simulink model "Copter_Plane_h3zh_sl_4a1rh"  (R2020b)
(part 2 of 3)

  use_sqrt_controller1 : DataStoreMemory  DataStoreName=use_sqrt_controller  ReadBeforeWriteMsg=warning  WriteAfterWriteMsg=warning  WriteAfterReadMsg=warning  InitialValue=use_sqrt_controller  ShowAdditionalParam=off  OutDataTypeStr=double
  vdot_filter1 : DataStoreMemory  DataStoreName=vdot_filter  ReadBeforeWriteMsg=warning  WriteAfterWriteMsg=warning  WriteAfterReadMsg=warning  InitialValue=vdot_filter  ShowAdditionalParam=off  OutDataTypeStr=double
  vel_desired1 : DataStoreMemory  DataStoreName=vel_desired  ReadBeforeWriteMsg=warning  WriteAfterWriteMsg=warning  WriteAfterReadMsg=warning  InitialValue=vel_desired  VectorParams1D=off  ShowAdditionalParam=off  OutDataTypeStr=double
  vel_dot1 : DataStoreMemory  DataStoreName=vel_dot  ReadBeforeWriteMsg=warning  WriteAfterWriteMsg=warning  WriteAfterReadMsg=warning  InitialValue=vel_dot  VectorParams1D=off  ShowAdditionalParam=off  OutDataTypeStr=double
  vel_error1 : DataStoreMemory  DataStoreName=vel_error  ReadBeforeWriteMsg=warning  WriteAfterWriteMsg=warning  WriteAfterReadMsg=warning  InitialValue=vel_error  VectorParams1D=off  ShowAdditionalParam=off  OutDataTypeStr=double
  vel_error_input1 : DataStoreMemory  DataStoreName=vel_error_input  ReadBeforeWriteMsg=warning  WriteAfterWriteMsg=warning  WriteAfterReadMsg=warning  InitialValue=vel_error_input  VectorParams1D=off  ShowAdditionalParam=off  OutDataTypeStr=double
  vel_forward_gain1 : DataStoreMemory  DataStoreName=vel_forward_gain  ReadBeforeWriteMsg=warning  WriteAfterWriteMsg=warning  WriteAfterReadMsg=warning  InitialValue=vel_forward_gain  VectorParams1D=off  ShowAdditionalParam=off  OutDataTypeStr=double
  vel_forward_integrator : DataStoreMemory  DataStoreName=vel_forward_integrator  ReadBeforeWriteMsg=warning  WriteAfterWriteMsg=warning  WriteAfterReadMsg=warning  InitialValue=vel_forward_integrator  VectorParams1D=off  ShowAdditionalParam=off  OutDataTypeStr=double
  vel_forward_last_pct1 : DataStoreMemory  DataStoreName=vel_forward_last_pct  ReadBeforeWriteMsg=warning  WriteAfterWriteMsg=warning  WriteAfterReadMsg=warning  InitialValue=vel_forward_last_pct  VectorParams1D=off  ShowAdditionalParam=off  OutDataTypeStr=double
  vel_forward_min_pitch1 : DataStoreMemory  DataStoreName=vel_forward_min_pitch  ReadBeforeWriteMsg=warning  WriteAfterWriteMsg=warning  WriteAfterReadMsg=warning  InitialValue=vel_forward_min_pitch  VectorParams1D=off  ShowAdditionalParam=off  OutDataTypeStr=double
  vel_forward_tail_tilt_max1 : DataStoreMemory  DataStoreName=vel_forward_tail_tilt_max  ReadBeforeWriteMsg=warning  WriteAfterWriteMsg=warning  WriteAfterReadMsg=warning  InitialValue=vel_forward_tail_tilt_max  VectorParams1D=off  ShowAdditionalParam=off  OutDataTypeStr=double
  vel_last1 : DataStoreMemory  DataStoreName=vel_last  ReadBeforeWriteMsg=warning  WriteAfterWriteMsg=warning  WriteAfterReadMsg=warning  InitialValue=vel_last  VectorParams1D=off  ShowAdditionalParam=off  OutDataTypeStr=double
  vel_target1 : DataStoreMemory  DataStoreName=vel_target  ReadBeforeWriteMsg=warning  WriteAfterWriteMsg=warning  WriteAfterReadMsg=warning  InitialValue=vel_target  VectorParams1D=off  ShowAdditionalParam=off  OutDataTypeStr=double
  vertAccLim1 : DataStoreMemory  DataStoreName=vertAccLim  ReadBeforeWriteMsg=warning  WriteAfterWriteMsg=warning  WriteAfterReadMsg=warning  InitialValue=vertAccLim  VectorParams1D=off  ShowAdditionalParam=off  OutDataTypeStr=double
  weathervane_gain1 : DataStoreMemory  DataStoreName=weathervane_gain  ReadBeforeWriteMsg=warning  WriteAfterWriteMsg=warning  WriteAfterReadMsg=warning  InitialValue=weathervane_gain  VectorParams1D=off  ShowAdditionalParam=off  OutDataTypeStr=double
  weathervane_last_output1 : DataStoreMemory  DataStoreName=weathervane_last_output  ReadBeforeWriteMsg=warning  WriteAfterWriteMsg=warning  WriteAfterReadMsg=warning  InitialValue=weathervane_last_output  VectorParams1D=off  ShowAdditionalParam=off  OutDataTypeStr=double
  weathervane_min_roll1 : DataStoreMemory  DataStoreName=weathervane_min_roll  ReadBeforeWriteMsg=warning  WriteAfterWriteMsg=warning  WriteAfterReadMsg=warning  InitialValue=weathervane_min_roll  VectorParams1D=off  ShowAdditionalParam=off  OutDataTypeStr=double
  yaw1 : DataStoreMemory  DataStoreName=yaw  ReadBeforeWriteMsg=warning  WriteAfterWriteMsg=warning  WriteAfterReadMsg=warning  InitialValue=yaw  VectorParams1D=off  ShowAdditionalParam=off  OutDataTypeStr=double
  yaw_factor1 : DataStoreMemory  DataStoreName=yaw_factor  ReadBeforeWriteMsg=warning  WriteAfterWriteMsg=warning  WriteAfterReadMsg=warning  InitialValue=yaw_factor  VectorParams1D=off  ShowAdditionalParam=off  OutDataTypeStr=double
  yaw_headroom1 : DataStoreMemory  DataStoreName=yaw_headroom  ReadBeforeWriteMsg=warning  WriteAfterWriteMsg=warning  WriteAfterReadMsg=warning  InitialValue=yaw_headroom  VectorParams1D=off  ShowAdditionalParam=off  OutDataTypeStr=double
  yaw_in1 : DataStoreMemory  DataStoreName=yaw_in  ReadBeforeWriteMsg=warning  WriteAfterWriteMsg=warning  WriteAfterReadMsg=warning  InitialValue=yaw_in  VectorParams1D=off  ShowAdditionalParam=off  OutDataTypeStr=double
  yaw_in_max : DataStoreMemory  DataStoreName=yaw_in_max  ReadBeforeWriteMsg=warning  WriteAfterWriteMsg=warning  WriteAfterReadMsg=warning  InitialValue=yaw_in_max  VectorParams1D=off  ShowAdditionalParam=off  OutDataTypeStr=double
  yaw_max_c2p1 : DataStoreMemory  DataStoreName=yaw_max_c2p  ReadBeforeWriteMsg=warning  WriteAfterWriteMsg=warning  WriteAfterReadMsg=warning  InitialValue=yaw_max_c2p  VectorParams1D=off  ShowAdditionalParam=off  OutDataTypeStr=double
  yaw_rate_max1 : DataStoreMemory  DataStoreName=yaw_rate_max  ReadBeforeWriteMsg=warning  WriteAfterWriteMsg=warning  WriteAfterReadMsg=warning  InitialValue=yaw_rate_max  VectorParams1D=off  ShowAdditionalParam=off  OutDataTypeStr=double
  yaw_t1 : Lookup_n-D  NumberOfTableDimensions=1  BreakpointsForDimension1=time_algo  Table=algo_yaw  InternalRulePriority=Speed  RndMeth=Simplest  InputSameDT=on
  z_accel_meas1 : DataStoreMemory  DataStoreName=z_accel_meas  ReadBeforeWriteMsg=warning  WriteAfterWriteMsg=warning  WriteAfterReadMsg=warning  InitialValue=z_accel_meas  VectorParams1D=off  ShowAdditionalParam=off  OutDataTypeStr=double
  Out1 : Outport  OutDataTypeStr=Bus: BUS_CTRL_Sevro_pwm
  wires:
  Gain15/1 -> Scope89/1
  Data Store Read75/1 -> Gain15/1
  Data Store Read77/1 -> Gain17/1
  Gain16/1 -> Scope90/1
  Data Store Read76/1 -> Gain16/1
  Gain17/1 -> Scope91/1
  Data Store Read2/1 -> Scope10/1
  Gain8/1 -> Scope13/1
  Gain3/1 -> Scope12/1
  Gain2/1 -> Scope11/1
  Data Store Read3/1 -> Gain2/1
  Data Store Read4/1 -> Gain3/1
  Data Store Read35/1 -> Gain8/1
  Data Store Read47/1 -> Demux/1
  Demux/1 -> Scope24/1
  Demux/2 -> Scope24/2
  Demux17/3 -> Scope14/3
  Demux17/2 -> Scope14/2
  Demux17/1 -> Scope14/1
  Data Store Read78/1 -> Demux17/1
  Data Store Read82/1 -> Scope39/1
  Data Store Read81/1 -> Scope30/1
  Data Store Read80/1 -> Scope23/1
  Data Store Read49/1 -> Scope47/1
  Data Store Read89/1 -> Scope63/1
  Data Store Read91/1 -> Scope69/1
  Data Store Read94/1 -> Scope6/2
  Data Store Read96/1 -> Scope16/2
  Data Store Read93/1 -> Scope18/2
  Data Store Read95/1 -> Scope132/1, Scope19/2
  Data Store Read97/1 -> Scope82/1
  Data Store Read98/1 -> Scope84/1
  Data Store Read99/1 -> Gain21/1
  Gain21/1 -> Scope107/2
  Data Store Read100/1 -> Gain22/1
  Gain22/1 -> Scope34/1, Scope4/1, Scope107/1
  Gain25/1 -> Scope35/1, Scope111/1
  Gain24/1 -> Scope111/2
  Data Store Read104/1 -> Gain24/1
  Data Store Read103/1 -> Scope36/1, Gain25/1
  Data Store Read105/1 -> Scope112/1
  Data Store Read106/1 -> Scope112/2
  Data Store Read5/1 -> Scope3/2, Scope1/1
  Data Store Read6/1 -> Scope3/1, Scope2/1
  Data Store Read8/1 -> Scope5/2
  Data Store Read7/1 -> Scope5/1, Scope4/2
  Data Store Read10/1 -> Scope8/1
  Data Store Read12/1 -> Scope109/1, Scope9/1
  Data Store Read13/1 -> Scope9/2
  Data Store Read14/1 -> Gain1/1
  Gain1/1 -> Scope8/2
  Data Store Read9/1 -> Scope15/1
  algo_throttle_dem/1 -> Data Store Write3/1
  Clock1/1 -> algo_pitch_dem/1, algo_k_aileron/1, algo_k_throttle/1, algo_k_rudder/1, algo_k_elevator/1
  algo_k_aileron/1 -> Gain61/1
  algo_k_elevator/1 -> Gain62/1
  algo_k_rudder/1 -> Gain63/1
  algo_k_throttle/1 -> Gain26/1
  Data Store Read17/1 -> Gain13/1
  Gain12/1 -> Scope41/3
  Gain13/1 -> Scope41/4
  Data Store Read16/1 -> Scope41/2, Scope42/2, Scope40/1
  Data Store Read/1 -> Scope42/1, Scope41/1, Scope/1
  Data Store Read15/1 -> Gain12/1
  Data Store Read18/1 -> Gain14/1
  Gain14/1 -> Scope112/3
  Data Store Read19/1 -> Scope43/1
  Data Store Read20/1 -> Scope43/2
  EAS_Algo/1 -> ?
  algo_curr_alt_0/1 -> Data Store Write19/1
  algo_curVelNED_2/1 -> Data Store Write25/1
  Data Store Read21/1 -> Gain18/1
  algo_pitch_dem/1 -> Scope38/1
  Gain18/1 -> Scope38/2
  Data Store Read23/1 -> Scope45/1
  Mux1/1 -> Gain69/1
  Gain30/1 -> Data Store Write30/1
  Gain32/1 -> Data Store Write42/1
  algo_remote_ct_st_throttle/1 -> Data Store Write40/1
  algo_roll_target_pilot/1 -> Gain10/1
  gx_f2/1 -> Gain19/1
  algo_current_loc_1/1 -> Mux2/2
  algo_curr_vel_2/1 -> Mux1/3
  algo_pitch_target_pilot/1 -> Gain11/1
  algo_remote_ct_st_yaw/1 -> Data Store Write45/1
  gy_f2/1 -> Gain32/1
  pitch_t1/1 -> Gain29/1
  algo_remote_ct_st_pitch/1 -> Data Store Write35/1
  ay_f2/1 -> Data Store Write31/1
  az_f2/1 -> Data Store Write36/1
  algo_curr_vel_0/1 -> Mux1/1
  algo_climb_rate_cms/1 -> Gain65/1
  algo_curr_vel_1/1 -> Mux1/2
  algo_curr_alt/1 -> Gain64/1
  ax_f2/1 -> Data Store Write32/1
  gz_f2/1 -> Gain33/1
  roll_t1/1 -> Gain30/1
  yaw_t1/1 -> Gain31/1
  Gain19/1 -> Data Store Write41/1
  Gain31/1 -> Data Store Write39/1
  Mux2/1 -> Gain/1
  Gain33/1 -> Data Store Write43/1
  algo_current_loc_0/1 -> Mux2/1
  Gain29/1 -> Data Store Write38/1
  algo_remote_ct_st_roll/1 -> Data Store Write8/1
  algo_curVelNED_1/1 -> Data Store Write5/1
  algo_curVelNED_0/1 -> Data Store Write4/1
  algo_throttle_upper/1 -> Scope66/1
  Data Store Read51/1 -> Demux1/1
  Data Store Read28/1 -> Scope58/2
  algo_rate_target_ang_vel_0/1 -> Gain6/1
  algo_z_accel_meas/1 -> Gain71/1
  algo_pos_target_0/1 -> Scope31/1
  Data Store Read33/1 -> Gain73/1
  Data Store Read53/1 -> Scope110/1, Scope37/2
  Data Store Read52/1 -> Scope32/2
  Data Store Read11/1 -> Gain53/1
  Data Store Read37/1 -> Gain89/1
  Data Store Read45/1 -> Gain4/1
  algo_vel_target_0/1 -> Scope25/1
  Clock5/1 -> algo_curr_pos_1/1, algo_curr_pos_0/1
  Gain5/1 -> Data Store Write7/1, Scope65/1
  Data Store Read50/1 -> Scope65/3
  algo_vel_desired_2/1 -> Scope26/1
  Gain6/1 -> Data Store Write/1, Scope59/1
  algo_rate_target_ang_vel_1/1 -> Gain7/1
  Demux1/1 -> Scope44/2
  algo_curr_pos_0/1 -> Scope44/1
  Clock6/1 -> algo_rate_target_ang_vel_2/1, algo_rate_target_ang_vel_1/1, algo_rate_target_ang_vel_0/1
  Data Store Read54/1 -> Scope60/2
  Demux1/2 -> Scope27/2
  Gain37/1 -> Scope61/1
  algo_vel_target_2/1 -> Gain66/1
  Clock12/1 -> algo_pitch_in/1
  algo_pos_target_1/1 -> Scope20/1
  Clock9/1 -> algo_roll_in/1
  Gain40/1 -> Scope64/2
  Data Store Read30/1 -> Scope56/2, Scope48/1
  Clock13/1 -> algo_yaw_in/1
  Clock3/1 -> algo_vel_target_1/1, algo_accel_target_1/1, algo_pos_target_1/1
  Clock10/1 -> algo_throttle_filter/1
  Data Store Read31/1 -> Scope29/2
  Data Store Read46/1 -> Scope59/3
  Data Store Read26/1 -> Derivative/1, Scope21/2
  algo_vel_target_1/1 -> Scope67/1
  Data Store Read44/1 -> Gain40/1
  Data Store Read25/1 -> Gain86/1
  Data Store Read42/1 -> Gain37/1
  Data Store Read24/1 -> Gain88/1
  Data Store Read22/1 -> Scope62/2, Scope110/2
  Data Store Read36/1 -> Gain91/1
  Gain39/1 -> Scope61/2
  Clock11/1 -> algo_pwm_out_4/1, algo_pwm_out_3/1, algo_pwm_out_2/1, algo_pwm_out_1/1
  Data Store Read43/1 -> Gain39/1
  Data Store Read1/1 -> Scope59/2
  algo_roll_in/1 -> Gain48/1
  algo_pwm_out_1/1 -> Scope46/1
  Data Store Read32/1 -> Scope33/2
  Data Store Read55/1 -> Scope65/2
  Clock8/1 -> algo_pos_target_0/1, algo_accel_target_0/1, algo_vel_target_0/1
  algo_pwm_out_2/1 -> Scope49/1
  algo_accel_target_1/1 -> Scope68/1
  Data Store Read29/1 -> Scope66/2
  algo_accel_target_2/1 -> Gain70/1
  Clock4/1 -> algo_throttle_upper/1, algo_throttle_lower/1, algo_limit_pos_up/1
  algo_throttle_lower/1 -> Scope58/1
  Clock7/1 -> algo_pos_target_2/1, algo_z_accel_meas/1, algo_accel_target_2/1, algo_vel_target_2/1, algo_vel_desired_2/1
  algo_yaw_in/1 -> Gain93/1
  algo_accel_target_0/1 -> Scope28/1
  algo_pitch_in/1 -> Gain92/1
  algo_limit_pos_up/1 -> Scope56/1
  algo_rate_target_ang_vel_2/1 -> Gain5/1
  Data Store Read41/1 -> Scope55/2
  Data Store Read38/1 -> Scope46/2
  Data Store Read34/1 -> Gain90/1
  Gain4/1 -> Scope64/1
  algo_curr_pos_1/1 -> Scope27/1
  algo_throttle_filter/1 -> Gain27/1
  algo_pwm_out_4/1 -> Scope55/1
  Data Store Read40/1 -> Scope50/2
  Data Store Read27/1 -> Derivative1/1, Scope22/2
  Data Store Read39/1 -> Scope49/2
  algo_pwm_out_3/1 -> Scope50/1
  Data Store Read48/1 -> Scope60/3
  Data Store Read56/1 -> Gain87/1
  Data Store Read57/1 -> Demux2/1
  Demux2/1 -> Scope17/1
  Demux2/2 -> Scope17/2
  Demux2/3 -> Scope17/3
  Gain7/1 -> Data Store Write6/1, Scope60/1
  algo_tail_tilt/1 -> Gain9/1
  Gain9/1 -> Data Store Write9/1
  Gain/1 -> Data Store Write33/1
  Gain10/1 -> Data Store Write34/1
  Gain11/1 -> Data Store Write37/1
  Data Store Read58/1 -> Demux3/1
  Data Store Read60/1 -> Scope53/1
  Demux3/1 -> Gain23/1
  Gain23/1 -> Scope53/2
  Demux3/2 -> Gain28/1
  Gain28/1 -> Scope70/1
  Data Store Read59/1 -> Scope70/2
  Data Store Read61/1 -> Scope71/1
  Data Store Read62/1 -> Scope71/2
  Data Store Read63/1 -> Scope72/2
  Data Store Read64/1 -> Scope52/1
  Data Store Read65/1 -> Scope71/3, Scope72/1
  EAS2TAS_Algo/1 -> Data Store Write18/1
  Gain34/1 -> Scope76/1
  Data Store Read69/1 -> Scope76/2
  Data Store Read68/1 -> Gain34/1
  Clock14/1 -> algo_weathervane_last_output/1
  algo_weathervane_last_output/1 -> Scope77/1
  Data Store Read70/1 -> Scope77/2
  Clock15/1 -> algo_attitude_target_euler_angle_2/1, algo_attitude_target_euler_angle_1/1, algo_attitude_target_euler_angle_0/1
  Data Store Read73/1 -> Gain35/1
  algo_attitude_target_euler_angle_2/1 -> Scope51/1
  Gain35/1 -> Scope51/2
  Data Store Read90/1 -> Scope87/1
  Data Store Read88/1 -> Scope87/2
  Data Store Read92/1 -> Scope88/2
  Data Store Read101/1 -> Scope88/1
  algo_flightTaskMode/1 -> Scope141/1, Data Type Conversion/1
  Data Type Conversion/1 -> Data Store Write12/1
  Data Store Read120/1 -> Demux4/1
  Data Store Read121/1 -> Gain49/1
  algo_attitude_target_euler_angle_1/1 -> Scope102/1
  Data Store Read124/1 -> Gain50/1
  algo_attitude_target_euler_angle_0/1 -> Scope103/1
  Gain49/1 -> Scope102/2
  Gain50/1 -> Scope103/2
  Data Store Read126/1 -> Scope105/2
  Data Store Read125/1 -> Scope104/2
  algo_attitude_target_euler_rate_0/1 -> Scope105/1
  algo_attitude_target_euler_rate_1/1 -> Scope104/1
  Data Store Read127/1 -> Scope106/2
  algo_attitude_target_euler_rate_2/1 -> Scope106/1
  Clock19/1 -> algo_attitude_target_euler_rate_0/1, algo_attitude_target_euler_rate_1/1, algo_attitude_target_euler_rate_2/1
  Data Store Read129/1 -> Gain51/1
  Gain51/1 -> Scope108/1, Scope109/2
  Data Store Read128/1 -> Scope108/2
  algo_heightCmd/1 -> Gain52/1
  Gain52/1 -> Data Store Write11/1
  algo_maxClimbSpeed/1 -> Data Store Write13/1
  algo_pos_target_2/1 -> Scope136/3, Scope7/1
  algo_turnCenterLL_0/1 -> Gain55/1
  algo_turnCenterLL_1/1 -> Gain56/1
  Gain55/1 -> Data Store Write14/1
  Gain56/1 -> Data Store Write15/1
  algo_prePathPoint_LLA_0/1 -> Gain57/1
  Gain57/1 -> Data Store Write16/1
  algo_prePathPoint_LLA_1/1 -> Gain58/1
  Gain58/1 -> Data Store Write17/1
  algo_curPathPoint_LLA_0/1 -> Gain59/1
  Gain59/1 -> Data Store Write20/1
  Gain60/1 -> Data Store Write21/1
  algo_curPathPoint_LLA_1/1 -> Gain60/1
  Gain61/1 -> Scope6/1
  Gain62/1 -> Scope16/1
  Gain63/1 -> Scope18/1
  Gain64/1 -> Data Store Write44/1
  Gain65/1 -> Data Store Write26/1
  Gain66/1 -> Scope32/1
  Data Store Read130/1 -> Scope115/1
  Clock16/1 -> algo_hgt_dem/1
  Data Store Read131/1 -> Gain67/1
  algo_hgt_dem/1 -> Scope116/1
  Gain67/1 -> Scope116/2
  Clock20/1 -> algo_nav_roll/1
  algo_nav_roll/1 -> Scope117/1
  Data Store Read132/1 -> Gain68/1
  Gain68/1 -> Scope117/2
  Clock21/1 -> algo_latAccDem1/1
  algo_latAccDem1/1 -> Scope118/1
  Data Store Read133/1 -> Scope118/2
  Data Store Read137/1 -> Scope122/1
  algo_nav_pitch_cd/1 -> Scope122/2, Data Store Write2/1
  algo_rollCmd/1 -> Data Store Write22/1
  Data Store Read138/1 -> Scope57/1
  Clock22/1 -> algo_curPosNED_1/1, algo_curPosNED_0/1
  Data Store Read140/1 -> Demux6/1
  Data Store Read141/1 -> Demux5/1
  Data Store Read139/1 -> Demux7/1
  Demux6/1 -> Scope123/1  "pre"
  Demux5/1 -> Scope123/2  "net"
  Demux6/2 -> Scope124/1
  Demux5/2 -> Scope124/2
  Demux7/2 -> Scope127/1, Scope124/3  "cur"
  algo_curPosNED_0/1 -> ?
  algo_curPosNED_1/1 -> ?
  Gain69/1 -> Data Store Write46/1
  Gain70/1 -> Scope37/1
  Gain71/1 -> Scope62/1
  Gain73/1 -> Scope26/2
  Gain53/1 -> Scope7/2
  algo_pos_target_2a/1 -> Gain75/1
  algo_vel_desired_2a/1 -> Gain74/1
  Gain74/1 -> Data Store Write24/1
  Gain75/1 -> Data Store Write23/1
  Data Store Read152/1 -> Scope130/1
  Data Store Read153/1 -> Scope131/1
  algo_arspeed/1 -> Scope131/2
  Clock23/1 -> algo_arspeed/1
  Data Store Read154/1 -> Scope133/1, Scope132/2
  Data Store Read155/1 -> Scope133/2
  Data Store Read157/1 -> Gain80/1
  Gain80/1 -> Scope134/2
  Data Store Read156/1 -> Scope134/1
  Gain81/1 -> Scope136/1
  Data Store Read162/1 -> Gain81/1
  Data Store Read163/1 -> Gain82/1
  Gain82/1 -> Scope136/2
  Data Store Read164/1 -> Scope137/1
  Data Store Read168/1 -> Demux8/1
  Demux8/1 -> Scope126/2  "cur"
  Demux7/1 -> Scope126/1, Scope123/3
  Demux8/2 -> Scope127/2  "cur"
  Gain86/1 -> Scope20/2
  Gain87/1 -> Scope67/2
  Gain88/1 -> Scope68/2
  Gain89/1 -> Scope31/2
  Gain90/1 -> Scope25/2
  Gain91/1 -> Scope28/2
  Clock17/1 -> algo_tail_tilt1/1
  algo_tail_tilt1/1 -> Scope101/2
  Data Store Read170/1 -> Scope101/1
  Clock24/1 -> algo_throttle_dem1/1
  algo_throttle_dem1/1 -> Scope139/1
  Data Store Read66/1 -> Scope139/2
  Data Store Read169/1 -> Scope140/1
  algo_plane_mode/1 -> Data Type Conversion1/1
  Data Type Conversion1/1 -> Data Store Write27/1, Scope142/1
  algo_flightControlMode/1 -> Data Type Conversion2/1
  Data Type Conversion2/1 -> Scope143/1, Data Store Write28/1
  algo_mode/1 -> Scope113/1, Ceil1/1
  Ceil1/1 -> Scope114/1, Data Store Write29/1
  Clock2/1 -> algo_hgt_dem1/1, algo_tail_tilt/1, yaw_t1/1, roll_t1/1, pitch_t1/1, gz_f2/1, gy_f2/1, gx_f2/1, az_f2/1, ay_f2/1, ax_f2/1, algo_current_loc_1/1, algo_current_loc_0/1, algo_curr_alt_0/1, algo_curr_alt/1, algo_curr_vel_1/1, algo_curVelNED_2/1, algo_curVelNED_0/1, EAS_Algo/1, EAS2TAS_Algo/1, algo_pitch_target_pilot/1, algo_roll_target_pilot/1, algo_climb_rate_cms/1, algo_remote_ct_st_roll/1, algo_remote_ct_st_throttle/1, algo_mode/1, algo_nav_pitch_cd/1, algo_plane_mode/1, algo_turnCenterLL_1/1, algo_curPathPoint_LLA_1/1, algo_curPathPoint_LLA_0/1, algo_prePathPoint_LLA_1/1, algo_prePathPoint_LLA_0/1, algo_vel_desired_2a/1, algo_pos_target_2a/1, algo_rollCmd/1, algo_turnCenterLL_0/1, algo_heightCmd/1, algo_flightControlMode/1, algo_flightTaskMode/1, algo_maxClimbSpeed/1, algo_throttle_dem/1, algo_remote_ct_st_pitch/1, algo_remote_ct_st_yaw/1, algo_arspeed1/1, algo_curVelNED_1/1, algo_curr_vel_0/1, algo_curr_vel_2/1
  Data Store Read167/1 -> Add2/2, Scope78/2
  Gain77/1 -> Scope128/3
  Data Store Read135/1 -> Scope120/1
  Data Store Read142/1 -> Gain72/1
  Data Store Read166/1 -> Add2/1, Add1/2
  Add/1 -> Gain84/1
  Data Store Read147/1 -> Gain78/1
  Gain85/1 -> Scope125/4
  Add1/1 -> Scope78/1
  Data Store Read145/1 -> Scope128/2
  Gain83/1 -> Scope125/1, Add/1
  Data Store Read143/1 -> Scope125/3, Add/3
  Data Store Read146/1 -> Gain77/1
  Gain84/1 -> Add1/1
  Gain72/1 -> Scope125/2, Add/2
  Data Store Read148/1 -> Scope129/2
  Gain78/1 -> Scope129/1
  Gain76/1 -> Scope128/1
  Data Store Read144/1 -> Gain76/1
  Gain79/1 -> Scope129/3
  Data Store Read134/1 -> Scope119/1
  Data Store Read149/1 -> Gain79/1
  Data Store Read136/1 -> Scope121/1
  Add2/1 -> Gain85/1
  Data Store Read71/1 -> Gain83/1
  Data Store Read158/1 -> Scope135/1
  Data Store Read160/1 -> Scope135/3
  Data Store Read159/1 -> Scope135/2
  Data Store Read161/1 -> Scope135/4
  Data Store Read150/1 -> Scope83/3  "I"
  Data Store Read85/1 -> Gain38/1
  Data Store Read151/1 -> Scope83/4
  Data Store Read86/1 -> Scope86/1
  Data Store Read84/1 -> Scope85/1
  Data Store Read83/1 -> Gain36/1
  Gain38/1 -> Scope85/2
  Data Store Read74/1 -> Scope83/1, Scope54/1  "P"
  Data Store Read165/1 -> Scope138/1
  Gain36/1 -> Scope81/1
  Data Store Read87/1 -> Gain41/1
  Gain41/1 -> Scope86/2
  Data Store Read79/1 -> Scope83/2, Scope80/1  "D"
  algo_hgt_dem1/1 -> Gain20/1
  Gain20/1 -> Data Store Write1/1
  ? -> Scope74/2
  Data Store Read72/1 -> Scope74/1
  algo_arspeed1/1 -> Data Store Write10/1
  Gain26/1 -> Scope19/1
  Clock25/1 -> algo_hgt_dem2/1
  algo_hgt_dem2/1 -> ?
  Gain27/1 -> Scope33/1
  Gain48/1 -> Scope21/1
  Gain92/1 -> Scope22/1
  Gain93/1 -> Scope29/1
  input_euler_angle_roll_pitch_euler_rate_yaw4/6(tail_tilt_o) -> Bus Assignment/7  "tail_tilt"
  input_euler_angle_roll_pitch_euler_rate_yaw4/3(k_rudder_o) -> Bus Assignment/4  "k_rudder"
  input_euler_angle_roll_pitch_euler_rate_yaw4/9(k_flap_o) -> Bus Assignment/10  "k_flap"
  input_euler_angle_roll_pitch_euler_rate_yaw4/1(k_alieron_o) -> Bus Assignment/2  "k_aileron"
  input_euler_angle_roll_pitch_euler_rate_yaw4/2(k_elevator_o) -> Bus Assignment/3  "k_elevator"
  input_euler_angle_roll_pitch_euler_rate_yaw4/7(pwm_out_o) -> Bus Assignment/8  "pwm_out"
  Bus Assignment/1 -> Out1/1
  input_euler_angle_roll_pitch_euler_rate_yaw4/4(k_aileronL_o) -> Bus Assignment/5  "k_rudderL"
  Constant/1 -> Bus Assignment/1
  input_euler_angle_roll_pitch_euler_rate_yaw4/8(pwm_tail_o) -> Bus Assignment/9  "pwm_tail"
  input_euler_angle_roll_pitch_euler_rate_yaw4/5(k_aileronR_o) -> Bus Assignment/6  "k_rudderR"
  Transpose1/1 -> Inertial to Body3/1
  Selector/1 -> Rotation Angles to Direction Cosine Matrix2/1
  Gain105/1 -> Scope159/2
  MATLAB Function14/1(forward) -> Gain113/1
  Gain94/1 -> Scope146/2
  Data Store Read195/1 -> MATLAB Function5/2(y_cmss)
  Data Store Read180/1 -> Gain114/1
  MATLAB Function14/2(right) -> Gain112/1
  Demux18/2 -> MATLAB Function14/2(y_cmss)
  Gain100/1 -> Scope148/1
  gn1/1 -> Add6/2
  MATLAB Function12/1(forward) -> Scope165/2
  Data Store Read186/1 -> Gain116/1
  Gain112/1 -> Scope153/2
  Data Store Read184/1 -> Mux8/1
  Gain103/1 -> Tan2/1
  Data Store Read218/1 -> MATLAB Function11/2(y_cmss)
  Gain95/1 -> Scope147/1
  Add6/1 -> Scope75/1, Demux18/1
  Gain109/1 -> Gain110/1
  Demux18/1 -> MATLAB Function14/1(x_cmss)
  Constant8/1 -> Mux8/3
  Rotation Angles to Direction Cosine Matrix2/1 -> Transpose1/1
  Data Store Read178/1 -> MATLAB Function10/2(y_cmss)
  Data Store Read183/1 -> Mux8/2
  Mux8/1 -> Selector/1
  Data Store Read176/1 -> MATLAB Function10/1(x_cmss)
  Gain113/1 -> Scope168/2
  Data Store Read215/1 -> MATLAB Function13/1(x_cmss)
  Data Store Read189/1 -> Gain117/1
  Gain114/1 -> Scope163/2
  Inertial to Body3/1 -> Add6/1, Scope169/1
  Mux6/1 -> Inertial to Body3/2
  Data Store Read212/1 -> MATLAB Function17/2(y_cmss)
  Data Store Read199/1 -> MATLAB Function9/2(y_cmss)
  Data Store Read219/1 -> Gain105/1
  Data Store Read220/1 -> Scope167/1
  Data Store Read210/1 -> MATLAB Function16/2(y_cmss)
  Data Store Read173/1 -> MATLAB Function5/1(x_cmss)
  MATLAB Function11/2(right) -> Scope158/1
  Gain102/1 -> Scope162/2, Scope159/1
  Data Store Read208/1 -> MATLAB Function15/1(x_cmss)
  Data Store Read206/1 -> Mux6/1
  Data Store Read182/1 -> Mux6/3
  Data Store Read211/1 -> MATLAB Function17/1(x_cmss)
  MATLAB Function10/2(right) -> Scope144/2, Scope160/1
  Data Store Read209/1 -> MATLAB Function15/2(y_cmss)
  MATLAB Function17/2(right) -> Scope161/1, Scope156/1, Scope144/1
  Data Store Read187/1 -> Gain94/1
  Data Store Read207/1 -> MATLAB Function16/1(x_cmss)
  MATLAB Function15/2(right) -> Scope161/2
  Data Store Read217/1 -> MATLAB Function11/1(x_cmss)
  Data Store Read216/1 -> MATLAB Function13/2(y_cmss)
  MATLAB Function16/2(right) -> Scope158/2
  MATLAB Function13/2(right) -> Scope160/2, Scope153/1, Scope157/1, Scope156/2
  Divide1/1 -> Scope157/2
  MATLAB Function5/1(forward) -> Scope154/1
  Data Store Read190/1 -> Gain95/1
  Data Store Read188/1 -> Gain96/1
  Data Store Read171/1 -> Scope164/2
  Data Store Read172/1 -> Scope164/1
  Data Store Read222/1 -> Gain104/1
  Data Store Read221/1 -> Scope162/1
  Data Store Read198/1 -> MATLAB Function9/1(x_cmss)
  Data Store Read200/1 -> Gain102/1
  Gain110/1 -> Divide1/2
  Gain116/1 -> Scope145/2
  Gain96/1 -> Scope147/2
  Data Store Read174/1 -> MATLAB Function12/1(x_cmss)
  Tan2/1 -> Divide1/1
  Data Store Read175/1 -> MATLAB Function12/2(y_cmss)
  Tan1/1 -> Gain109/1
  Gain107/1 -> Scope151/2
  Data Store Read214/1 -> Gain103/1
  Gain106/1 -> Gain107/1
  MATLAB Function9/1(forward) -> Scope152/2, Scope151/1, Scope168/1, Scope166/1, Scope155/2
  Data Store Read203/1 -> MATLAB Function8/2(y_cmss)
  Data Store Read205/1 -> MATLAB Function7/2(y_cmss)
  Gain101/1 -> Tan/1
  MATLAB Function8/1(forward) -> Scope154/2
  MATLAB Function6/1(forward) -> Scope165/1, Scope152/1, Scope150/1
  Data Store Read194/1 -> Gain100/1
  Data Store Read201/1 -> Gain101/1
  MATLAB Function7/1(forward) -> Scope150/2, Scope155/1
  Data Store Read213/1 -> Gain108/1
  Data Store Read202/1 -> MATLAB Function8/1(x_cmss)
  Data Store Read196/1 -> MATLAB Function6/1(x_cmss)
  Data Store Read197/1 -> MATLAB Function6/2(y_cmss)
  Gain108/1 -> Tan1/1
  Gain98/1 -> Scope149/1
  Tan/1 -> Gain106/1
  Data Store Read192/1 -> Gain98/1
  Gain115/1 -> Scope145/1
  Gain117/1 -> Scope146/1
  Data Store Read204/1 -> MATLAB Function7/1(x_cmss)
  Gain99/1 -> Scope148/2
  Gain97/1 -> Scope149/2
  Data Store Read185/1 -> Gain115/1
  Data Store Read191/1 -> Gain97/1
  Data Store Read181/1 -> Mux6/2
  Gain104/1 -> Scope167/2, Scope163/1
  Data Store Read193/1 -> Gain99/1
  Derivative/1 -> Scope73/1
  Derivative1/1 -> Scope79/1
  Constant1/1 -> Divide2/1
  Data Store Read67/1 -> Divide2/2
  Divide2/1 -> Scope93/1, Add3/1
  Data Store Read102/1 -> Scope93/2, Add3/2
  Add3/1 -> Scope92/1
  Data Store Read107/1 -> Scope92/2
